simulink model "StdAnimation_Test"  (R2020b)
settings: configuration reference "VLS_SIL_Configuration" (kept outside this file)
settings Model: DataDictionary=StdAnimation_TestingDD.sldd  PauseTimes=12.7  Creator=mchawa  LastModifiedBy=oashraf
settings ConfigSetRef: SourceName=VLS_SIL_Configuration

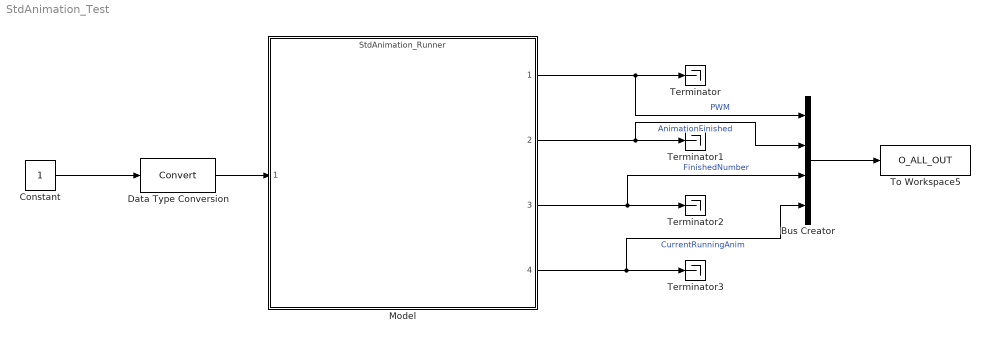
== system StdAnimation_Test ==
  Bus Creator : BusCreator  Inputs=4
  Constant : Constant
  Data Type Conversion : DataTypeConversion  RndMeth=Nearest
  Model : ModelReference  ModelNameDialog=StdAnimation_Runner.slx  SimulationMode=Normal  ModelReferenceVersion=1.77
  Terminator{,1..3} (4 alike) : Terminator
  To Workspace5 : ToWorkspace  VariableName=O_ALL_OUT  SaveFormat=Timeseries  SampleTime=-1
      settings: Save2DSignal=2-D array (concatenate along first dimension)
  wires:
  Model/1 -> Bus Creator/1, Terminator/1  "PWM"
  Model/2 -> Bus Creator/2, Terminator1/1  "AnimationFinished"
  Model/3 -> Bus Creator/3, Terminator2/1  "FinishedNumber"
  Model/4 -> Bus Creator/4, Terminator3/1  "CurrentRunningAnim"
  Bus Creator/1 -> To Workspace5/1
  Data Type Conversion/1 -> Model/1
  Constant/1 -> Data Type Conversion/1
